simulink model "polytrajD3"  (R2020b)
settings: Solver=VariableStepAuto  StartTime=0.0  StopTime=10.0  RelTol=1e-3
libraries: simulink x1
settings Model: Creator=mstra  LastModifiedBy=mstra

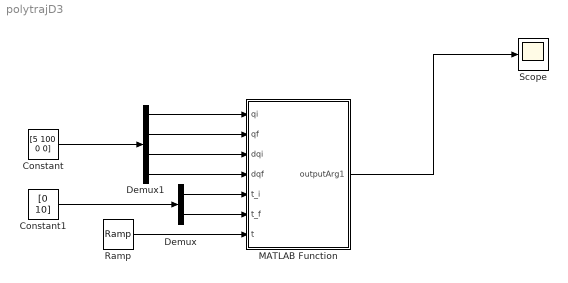
== system polytrajD3 ==
  Constant : Constant  Value=[5 100 0 0]
  Constant1 : Constant  Value=[0 10]
  Demux : Demux  Outputs=2
  Demux1 : Demux
  MATLAB Function : MATLAB Function  TreatAsAtomicUnit=on
  Ramp : simulink/Sources/Ramp  slope=1  start=0  InitialOutput=0
  Scope : Scope
  wires:
  Demux/1 -> MATLAB Function/5(t_i)
  Demux/2 -> MATLAB Function/6(t_f)
  Demux1/1 -> MATLAB Function/1(qi)
  Demux1/2 -> MATLAB Function/2(qf)
  Demux1/3 -> MATLAB Function/3(dqi)
  Demux1/4 -> MATLAB Function/4(dqf)
  Constant1/1 -> Demux/1
  Constant/1 -> Demux1/1
  Ramp/1 -> MATLAB Function/7(t)
  MATLAB Function/1(outputArg1) -> Scope/1

== matlab function polytrajD3/MATLAB Function ==
  data: qi input; outputArg1 output; qf input; dqi input; dqf input; t_i input; t_f input; t input
function outputArg1  = poly_traj_D3(qi, qf ,dqi ,dqf ,t_i ,t_f, t)
%makes polynomial from inputs

v = [qi dqi qf dqf]';
A = [1 t_i t_i^2 t_i^3; 0 1 2*t_i 3*t_i^2; 1 t_f t_f^2 t_f^3; 0 1 2*t_f 3*t_f^2];
% invert to get the coefficients
a = inv(A)*v;
% trying the matrix way
q = qi + dqi*(t-t_i) + a(3,1)*(t-t_i)^2 + a(4,1)*(t-t_i)^3;
% return position at t
outputArg1 = q;

end
